simulink model "regler_antiwindup_mdl"  (R2013b)
settings: Solver=ode45  StartTime=0.0  StopTime=0.5  RelTol=1e-3
values from neighbouring files (symbols this model uses):
  g_antiwindup = 1    [regler_antiwindup.m]
  K = 0.05    [regler_antiwindup.m]
  Kg = K / (K*K + a*R)    (= 16.6666666667)    [regler_antiwindup.m]
  Kp = 1    [regler_antiwindup.m]
  mmax = 0.00    (= 0)    [regler_antiwindup.m]
  R = 0.5    [regler_antiwindup.m]
  tau = J*R / (K*K + a*R)    (= 0.0416666666667)    [regler_antiwindup.m]
  Ti = tau    (= 0.0416666666667)    [regler_antiwindup.m]
settings Model: Creator=daniw  LastModifiedBy=daniw
settings DataIOCC: LimitDataPoints=off

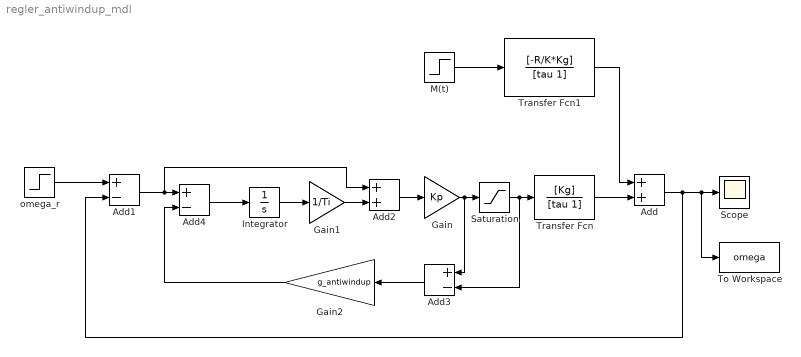
== system regler_antiwindup_mdl ==
  Add : Sum
  Add1 : Sum  Inputs=+-
  Add2 : Sum
  Add3 : Sum  Inputs=+-
  Add4 : Sum  Inputs=+-
  Gain : Gain  Gain=Kp
  Gain1 : Gain  Gain=1/Ti
  Gain2 : Gain  Gain=g_antiwindup
  Integrator : Integrator
  M(t) : Step  Time=2  After=mmax  SampleTime=0
  Saturation : Saturate  UpperLimit=10  LowerLimit=-10
  Scope : Scope
  To Workspace : ToWorkspace  VariableName=omega  SampleTime=-1  SaveFormat=Structure With Time
  Transfer Fcn : TransferFcn  Numerator=[Kg]  Denominator=[tau 1]
  Transfer Fcn1 : TransferFcn  Numerator=[-R/K*Kg]  Denominator=[tau 1]
  omega_r : Step  Time=0.1  Before=50  After=100  SampleTime=0
  wires:
  M(t)/1 -> Transfer Fcn1/1
  omega_r/1 -> Add1/1
  Add/1 -> Add1/2, To Workspace/1, Scope/1
  Transfer Fcn/1 -> Add/2
  Transfer Fcn1/1 -> Add/1
  Gain/1 -> Add3/1, Saturation/1
  Add1/1 -> Add4/1, Add2/1
  Integrator/1 -> Gain1/1
  Add2/1 -> Gain/1
  Gain1/1 -> Add2/2
  Saturation/1 -> Add3/2, Transfer Fcn/1
  Add3/1 -> Gain2/1
  Gain2/1 -> Add4/2
  Add4/1 -> Integrator/1
